simulink model "teeth"  (R2018a)
settings: Solver=FixedStepDiscrete  StartTime=0.0  StopTime=5  FixedStep=1e-5  RelTol=1e-3
InitFcn:
  | mbd_pnt_consistency_checks(bdroot(gcs));
undefined symbols (not defined in the file): AN, B, B14, C10, J, P9, PCR, R5, T12, T13
libraries: mbd_pnt_ec_toolbox x4, dspswit3 x1
settings Model: Creator=oolonthegreat  LastModifiedBy=oolonthegreat
settings DataIOCC: ExternalInput=off  InitialState=off  SaveOutput=off  SignalLogging=off  SaveTime=off
settings OptimizationCC: DefaultParameterBehavior=Inlined  EnhancedBackFolding=on  PassReuseOutputArgsAs=Individual arguments  OptimizeBlockOrder=speed  DifferentSizesBufferReuse=on  OptimizationCustomize=off
settings DebuggingCC: InheritedTsInSrcMsg=none  SingleTaskRateTransMsg=error  ParameterTunabilityLossMsg=error  UnconnectedInputMsg=error  UnconnectedOutputMsg=error  UnconnectedLineMsg=error  UnknownTsInhSupMsg=error
settings HardwareCC: ProdBitPerPointer=32  ProdBitPerSizeT=32  ProdBitPerPtrDiffT=32  ProdLargestAtomicInteger=Long  ProdLargestAtomicFloat=Double  ProdEndianess=BigEndian  ProdWordSize=32  ProdHWDeviceType=Motorola PowerPC
settings SFSimCC: MATLABDynamicMemAlloc=off
settings RTWCC: SystemTargetFile=mbd_pnt.tlc  MakeCommand=mbd_pnt_make_rtw COPY_MDLREF_INCLUDES=0  TemplateMakefile=mbd_pnt.tmf  PostCodeGenCommand=mbd_pnt_analyzegencode(buildInfo)  Description=Model Based Design Toolbox MPC574xP Code Generation Target  GenerateReport=on  IncludeHyperlinkInReport=on  LaunchReport=on  GenerateTraceInfo=on  GenerateTraceReport=on  GenerateTraceReportSl=on  GenerateTraceReportSf=on  GenerateTraceReportEml=on
settings CodeAppCC: ForceParamTrailComments=on  IgnoreCustomStorageClasses=off  OperatorAnnotations=on  SimulinkDataObjDesc=on  SFDataObjDesc=on  InsertBlockDesc=on
settings STFCustomTargetCC: TargetLangStandard=C99 (ISO)  MultiwordLength=256  CombineOutputUpdateFcns=on  SuppressErrorStatus=on  ERTCustomFileBanners=on  SupportContinuousTime=off  SupportNonInlinedSFcns=off  RemoveResetFunc=on  MATLABClassNameForMDSCustomization=Simulink.SoftwareTarget.ERTCustomization  GRTInterface=off  SystemTargetFile=mbd_pnt.tlc
settings ERTTargetCC: TargetLangStandard=C99 (ISO)  ParMdlRefBuildCompliant=off  CompOptLevelCompliant=off  ConcurrentExecutionCompliant=off  SuppressErrorStatus=on  ModelStepFunctionPrototypeControlCompliant=off  CPPClassGenCompliant=off  UseToolchainInfoCompliant=off  InlinedParameterPlacement=NonHierarchical  ERTCustomFileTemplate=example_file_process.tlc

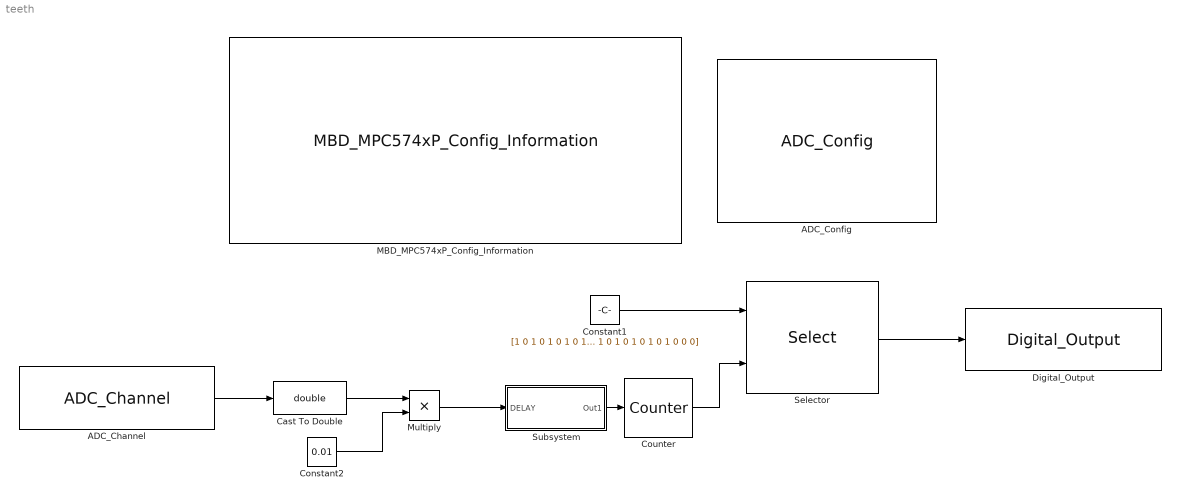
== system teeth ==
  ADC_Channel : mbd_pnt_ec_toolbox/MPC574xP/Motor Control Blocks/ADC_Channel  adc_unit=1  adc_chan0=PCR[23] : B[7] : 43 : 51 : R5 : AN[0]  adc_chan1=PCR[76] : E[12] : 67 : 78 : T12 : AN[6]  adc_chan2=PCR[150] : J[6] : [---] : 65 : P9 : AN[1]  adc_chan3=PCR[64] : E[0] : 68 : 79 : T13 : AN[4]  simulate=off  interrupt=off  adc_mode=Normal  adc_presample=off  pcrNum=76
      settings: SourceProductName=Model Based Design Toolbox for MPC574xP
  ADC_Config : mbd_pnt_ec_toolbox/MPC574xP/Motor Control Blocks/ADC_Config  adc_unit=1  adc_ctu=off  adc_owr=on  adc_wls=0: Left  adc_clk=on  adc_ack=on  adc_edglev=0: Edge  adc_trgen=off  adc_edge=off  adc_ctr0_samp=22  adc_ctr1_samp=11  adc_pscr_preval0=00: AGND_3V  adc_pscr_preconv=off  adc_calbist_admode=110: 12-bit operating mode (high accuracy)  adc_calbist_tsamp=00: 22 cycles of ADC clk  adc_calbist_nrsmpl=01: 32 samples  adc_calbist_avgen=on
      settings: SourceProductName=Model Based Design Toolbox for MPC574xP
  Cast To Double : DataTypeConversion  OutDataTypeStr=double
  Constant1 : Constant  Value=[1 0 1 0 1 0 1 0 1 0 1 0 1 0 1 0 1 0 1 0 1 0 1 0 1 0 1 0 1 0 0 0]  OutDataTypeStr=boolean
  Constant2 : Constant  Value=0.01
  Counter : dspswit3/Counter  Direction=Up  CountEvent=Rising edge  CounterSize=User defined  MaxCount=31  InitialCount=0  Output=Count  HitValue=32  ResetInput=off  SamplesPerFrame=1  Ts=1  CntDtype=double  HitDtype=Logical
  Digital_Output : mbd_pnt_ec_toolbox/MPC574xP/Peripheral Interface Blocks/Digital_Output  gpio_outputs="42   : C10 :  [111] : [136] : [B14]"  pinNum=[111]  pcrNum=42
      settings: SourceProductName=Model Based Design Toolbox for MPC574xP
  MBD_MPC574xP_Config_Information : mbd_pnt_ec_toolbox/MPC574xP/MBD_MPC574xP_Config_Information  disp_str=|  config_params=[]
      | System Clock : 200 MHz
      | Target : MPC5744P
      | Package : 144LQFP
      | XTAL Freq : 40 MHz
      | Compiler : S32 Design Studio
      | Target Type : FLASH
      | Global Interrupt Priority : 8
      | System Tick Interrupt Priority : 12
      | Freemaster : Serial1 (115200 Kbits)
      | Download Code after build : (COM5,115200)
      settings: SourceProductName=Model Based Design Toolbox for MPC574xP
  Multiply : Product
  Selector : Selector  IndexMode=Zero-based  InputPortWidth=32  IndexOptions=Index vector (port)  Indices=[1 3]  OutputSizes=1
  Subsystem : Subsystem
  wires:
  Counter/1 -> Selector/2
  Constant1/1 -> Selector/1
  Constant2/1 -> Multiply/2
  ADC_Channel/1 -> Cast To Double/1
  Multiply/1 -> Subsystem/1(DELAY)
  Cast To Double/1 -> Multiply/1
  Selector/1 -> Digital_Output/1
  Subsystem/1(Out1) -> Counter/1

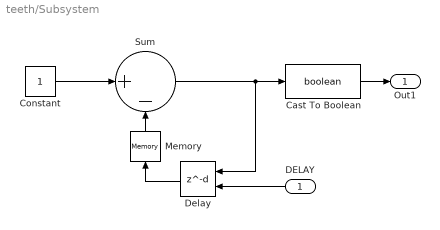
== system teeth/Subsystem ==
  DELAY : Inport
  Cast To Boolean : DataTypeConversion  OutDataTypeStr=boolean
  Constant : Constant  OutDataTypeStr=double
  Delay : Delay  DelayLengthSource=Input port
      settings: InputPortMap=u0,p1
  Memory : Memory
  Sum : Sum  Inputs=|+-  OutDataTypeStr=double
  Out1 : Outport
  wires:
  Constant/1 -> Sum/1
  Sum/1 -> Cast To Boolean/1, Delay/1
  Delay/1 -> Memory/1
  DELAY/1 -> Delay/2
  Memory/1 -> Sum/2
  Cast To Boolean/1 -> Out1/1
